simulink model "me132Hw1Q7_ClosedLoopControl"  (R2021a)
settings: Solver=VariableStepAuto  StartTime=0.0  StopTime=time_end  MaxStep=0.1  RelTol=1e-3
values from neighbouring files (symbols this model uses):
  c = 1    [hw1Q6.m]    (also in hw1Q7.m)
  k = 1.1    [hw1Q6.m]    (also in hw1Q7.m)
  m = 1    [hw1Q6.m]    (also in hw1Q7.m)
settings Model: Creator=kaiyu  LastModifiedBy=kaiyu

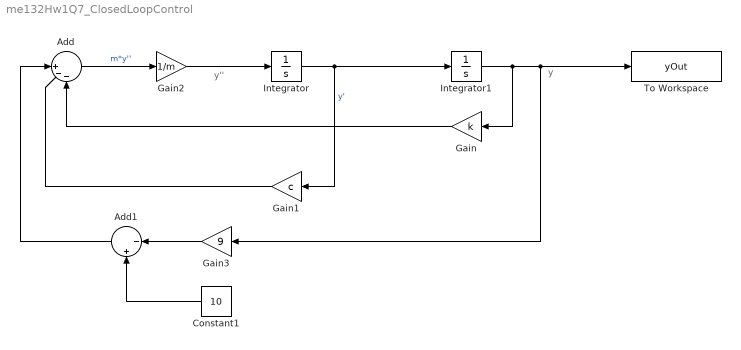
== system me132Hw1Q7_ClosedLoopControl ==
  note: y''
  note: y
  Add : Sum  Inputs=||+--
  Add1 : Sum  Inputs=||-|+
  Constant1 : Constant  Value=10
  Gain : Gain  Gain=k
  Gain1 : Gain  Gain=c
  Gain2 : Gain  Gain=1/m
  Gain3 : Gain  Gain=9
  Integrator : Integrator
  Integrator1 : Integrator
  To Workspace : ToWorkspace  VariableName=yOut  SaveFormat=Timeseries  SampleTime=-1
  wires:
  Gain2/1 -> Integrator/1
  Gain1/1 -> Add/2
  Gain/1 -> Add/3
  Integrator1/1 -> Gain/1, Gain3/1, To Workspace/1
  Integrator/1 -> Gain1/1, Integrator1/1  "y'"
  Add/1 -> Gain2/1  "m*y''"
  Gain3/1 -> Add1/1
  Constant1/1 -> Add1/2
  Add1/1 -> Add/1
